simulink model "skewSine"  (R2018b)
settings: Solver=FixedStepAuto  StartTime=0.0  StopTime=50  FixedStep=ts  RelTol=1e-3
undefined symbols (not defined in the file or in its folder): seed, sp_ts, tm
settings Model: Creator=wout7  LastModifiedBy=wout7

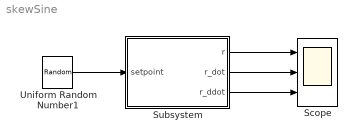
== system skewSine ==
  Scope : Scope  NumInputPorts=3
  Subsystem : Subsystem
  Uniform Random Number1 : UniformRandomNumber  Minimum=-50*pi/180  Maximum=50*pi/180  Seed=seed  SampleTime=sp_ts
  wires:
  Uniform Random Number1/1 -> Subsystem/1(setpoint)
  Subsystem/1(r) -> Scope/1
  Subsystem/2(r_dot) -> Scope/2
  Subsystem/3(r_ddot) -> Scope/3

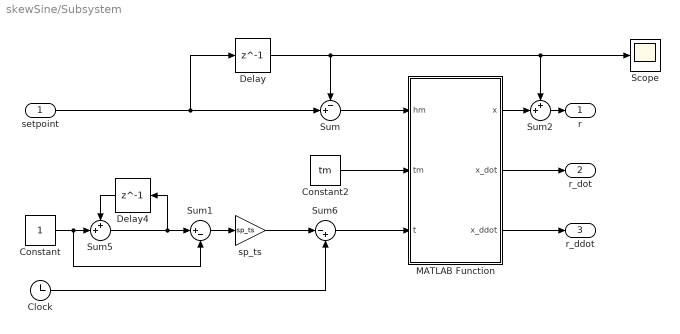
== system skewSine/Subsystem ==
  setpoint : Inport
  Clock : Clock
  Constant : Constant  SampleTime=sp_ts
  Constant2 : Constant  Value=tm  SampleTime=sp_ts
  Delay : Delay  DelayLength=1  InitialCondition=0  SampleTime=sp_ts
  Delay4 : Delay  DelayLength=1  InitialCondition=0  SampleTime=sp_ts
  MATLAB Function : MATLAB Function  TreatAsAtomicUnit=on
  Scope : Scope
  Sum : Sum  Inputs=-+|
  Sum1 : Sum  Inputs=|+-
  Sum2 : Sum  Inputs=++|
  Sum5 : Sum  Inputs=++|
  Sum6 : Sum  Inputs=|-+
  sp_ts : Gain  Gain=sp_ts
  r : Outport
  r_dot : Outport  Port=2
  r_ddot : Outport  Port=3
  wires:
  Constant2/1 -> MATLAB Function/2(tm)
  MATLAB Function/1(x) -> Sum2/2
  Delay4/1 -> Sum5/1
  Sum/1 -> MATLAB Function/1(hm)
  setpoint/1 -> Delay/1, Sum/2
  Sum2/1 -> r/1
  Sum5/1 -> Sum1/1, Delay4/1
  Constant/1 -> Sum1/2, Sum5/2
  MATLAB Function/3(x_ddot) -> r_ddot/1
  Clock/1 -> Sum6/2
  Sum6/1 -> MATLAB Function/3(t)
  sp_ts/1 -> Sum6/1
  MATLAB Function/2(x_dot) -> r_dot/1
  Delay/1 -> Sum2/1, Scope/1, Sum/1
  Sum1/1 -> sp_ts/1

== matlab function skewSine/Subsystem/MATLAB Function ==
  settings: updateMethod=DISCRETE  sampleTime=ts
  data: hm input; x output; tm input; t input; x_dot output; x_ddot output
function [x,x_dot,x_ddot] = skewSine(hm,tm,t)

if (t>=0) && (t<=tm)
    x      = hm/tm*t - hm/(2*pi)*sin(2*pi/tm*t);
    x_dot  = hm/tm - hm/tm*cos(2*pi/tm*t);
    x_ddot = 2*pi*hm/(tm^2)*sin(2*pi/tm*t);
else
    x      = hm;
    x_dot  = 0;
    x_ddot = 0;
end
